simulink model "ipLinkRec2"  (Simulink 7.4)
settings: Solver=FixedStepDiscrete  StartTime=0.0  StopTime=inf  FixedStep=1  RelTol=1e-3
settings Model: Creator=tyler  LastModifiedBy=tyler
settings RTWCC: SystemTargetFile=nrt.tlc  TemplateMakefile=nrt_unix.tmf  Description=Nokia Real-Time Target  ProcessScript=nrt_make_rtw_hook
settings STFCustomTargetCC: ModelReferenceCompliant=off  GeneratePreprocessorConditionals=Disable all  MatFileLogging=on  SystemTargetFile=nrt.tlc
settings GRTTargetCC: ModelReferenceCompliant=off  ParMdlRefBuildCompliant=off  CompOptLevelCompliant=off
settings CustomProperty: DataType=string  Value=-lm -ldl
settings EnumStrPairs: String=PC

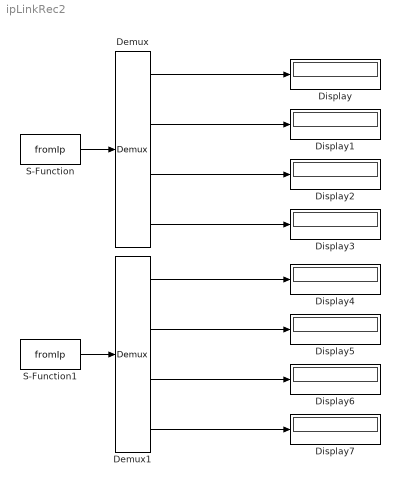
== system ipLinkRec2 ==
  Demux : Demux
  Demux1 : Demux
  Display{,1..7} (8 alike) : Display
  S-Function : S-Function  FunctionName=fromIp  Parameters='6665' 0  EnableBusSupport=off
  S-Function1 : S-Function  FunctionName=fromIp  Parameters='6666' 3  EnableBusSupport=off
  wires:
  S-Function/1 -> Demux/1
  Demux/1 -> Display/1
  Demux/2 -> Display1/1
  Demux/3 -> Display2/1
  Demux/4 -> Display3/1
  S-Function1/1 -> Demux1/1
  Demux1/1 -> Display4/1
  Demux1/2 -> Display5/1
  Demux1/3 -> Display6/1
  Demux1/4 -> Display7/1
